simulink model "simulink_model"  (R2019b)
settings: Solver=VariableStepAuto  StartTime=0.0  StopTime=30  RelTol=1e-3
libraries: simulink x1
settings Model: Creator=Ivan  LastModifiedBy=Ivan

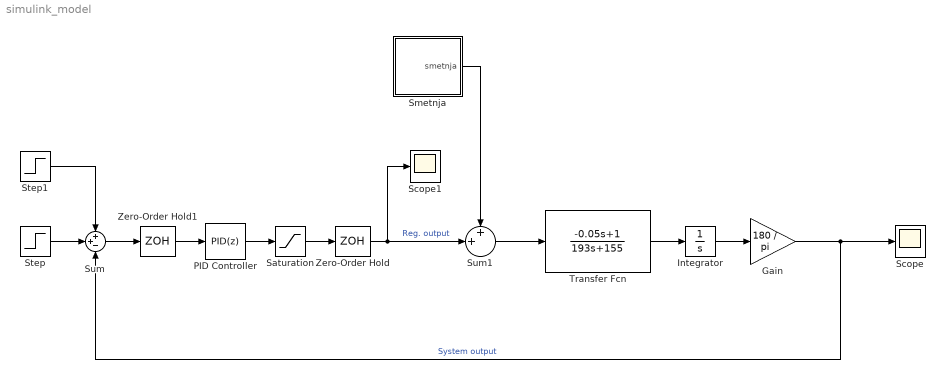
== system simulink_model ==
  Gain : Gain  Gain=180 / pi
  Integrator : Integrator
  PID Controller : simulink/Continuous/PID Controller  Controller=PID  Form=Parallel  TimeDomain=Discrete-time  SampleTime=0.1  IntegratorMethod=Forward Euler  FilterMethod=Forward Euler  ControllerParametersSource=internal  P=17  I=0  D=10  UseFilter=on  N=5  TunerSelectOption=Transfer Function Based (PID Tuner App)  InitialConditionSource=internal  InitialConditionForIntegrator=0  InitialConditionForFilter=0  DifferentiatorICPrevScaledInput=0  ExternalReset=none  TrackingMode=off  Kt=1  LimitOutput=off  UpperSaturationLimit=inf  LowerSaturationLimit=-inf  LinearizeAsGain=on  AntiWindupMode=none  Kb=1  POutMin=[]  POutMax=[]  IOutMin=[]  IOutMax=[]  DOutMin=[]  DOutMax=[]  NOutMin=[]  NOutMax=[]  SumOutMin=[]  SumOutMax=[]  SaturationOutMin=[]  SaturationOutMax=[]  PParamMin=[]  PParamMax=[]  IParamMin=[]  IParamMax=[]  DParamMin=[]  DParamMax=[]  NParamMin=[]  NParamMax=[]  KbParamMin=[]  KbParamMax=[]  KtParamMin=[]  KtParamMax=[]  KbOutMin=[]  KbOutMax=[]  KtOutMin=[]  KtOutMax=[]  IntegratorOutMin=[]  IntegratorOutMax=[]  FilterOutMin=[]  FilterOutMax=[]  SumI1OutMin=[]  SumI1OutMax=[]  SumI2OutMin=[]  SumI2OutMax=[]  SumI3OutMin=[]  SumI3OutMax=[]  SumI4OutMin=[]  SumI4OutMax=[]  SumDOutMin=[]  SumDOutMax=[]  DifferentiatorOutMin=[]  DifferentiatorOutMax=[]  FilterDiffOutCoefMin=[]  FilterDiffOutCoefMax=[]  ReciprocalOutMin=[]  ReciprocalOutMax=[]  SumDenOutMin=[]  SumDenOutMax=[]  SumNumOutMin=[]  SumNumOutMax=[]  DivideOutMin=[]  DivideOutMax=[]  IntegratorContinuousStateAttributes=''  IntegratorStateMustResolveToSignalObject=off  IntegratorRTWStateStorageClass=Auto  FilterContinuousStateAttributes=''  FilterStateMustResolveToSignalObject=off  FilterRTWStateStorageClass=Auto  ParallelPVariant=InternalParameters  IdealPVariant=Disabled  IVariant=InternalParameters  DVariant=InternalParameters  IntegratorVariant=Continuous  SatVariant=Disabled  AWVariant=Passthrough  PCopyVariant=Disabled  TRVariant=Disabled  FdbkBlocksVariant=Forward  IdealPFdbkVariant=Disabled  SatFdbkVariant=Disabled  DerivativeFilterVariant=ContFilter  NVariant=InternalParameters  NCopyVariant=Disabled  FilterICVariant=InternalICsFilter  IntegratorICVariant=InternalICs  ExternalResetVariant=Disabled  TRSumVariant=Passthrough  SumFdbkVariant=Disabled  SumVariant=Sum_PID
  Saturation : Saturate  UpperLimit=255  LowerLimit=-255
  Scope : Scope
  Scope1 : Scope
  Smetnja : Subsystem
  Step : Step  Time=0  After=50  SampleTime=0
  Step1 : Step  Time=20  After=-70  SampleTime=0
  Sum : Sum  Inputs=++-
  Sum1 : Sum  Inputs=++|
  Transfer Fcn : TransferFcn  Numerator=[-0.05 1]  Denominator=[193 155]
  Zero-Order Hold : ZeroOrderHold  SampleTime=0.1
  Zero-Order Hold1 : ZeroOrderHold  SampleTime=0.1
  wires:
  Transfer Fcn/1 -> Integrator/1
  PID Controller/1 -> Saturation/1
  Saturation/1 -> Zero-Order Hold/1
  Integrator/1 -> Gain/1
  Gain/1 -> Sum/3, Scope/1  "System output"
  Sum1/1 -> Transfer Fcn/1
  Zero-Order Hold/1 -> Scope1/1, Sum1/2  "Reg. output"
  Sum/1 -> Zero-Order Hold1/1
  Zero-Order Hold1/1 -> PID Controller/1
  Smetnja/1(smetnja) -> Sum1/1
  Step/1 -> Sum/2
  Step1/1 -> Sum/1

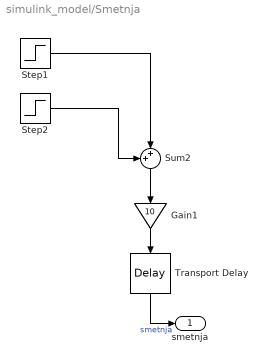
== system simulink_model/Smetnja ==
  Gain1 : Gain  Gain=10
  Step1 : Step  Time=3  SampleTime=0
  Step2 : Step  Time=4  After=-1  SampleTime=0
  Sum2 : Sum  Inputs=++|
  Transport Delay : TransportDelay  DelayTime=10  BufferSize=10240
  smetnja : Outport
  wires:
  Sum2/1 -> Gain1/1
  Step1/1 -> Sum2/2
  Step2/1 -> Sum2/1
  Gain1/1 -> Transport Delay/1
  Transport Delay/1 -> smetnja/1  "smetnja"
